simulink model "AcasXuClosedLoop"  (R2019b)
settings: Solver=VariableStepAuto  StartTime=0.0  StopTime=15.0  RelTol=1e-3
libraries: neural x312, simulink x2
(part 1 of 17)
settings Model: Creator=manzand  LastModifiedBy=manzand

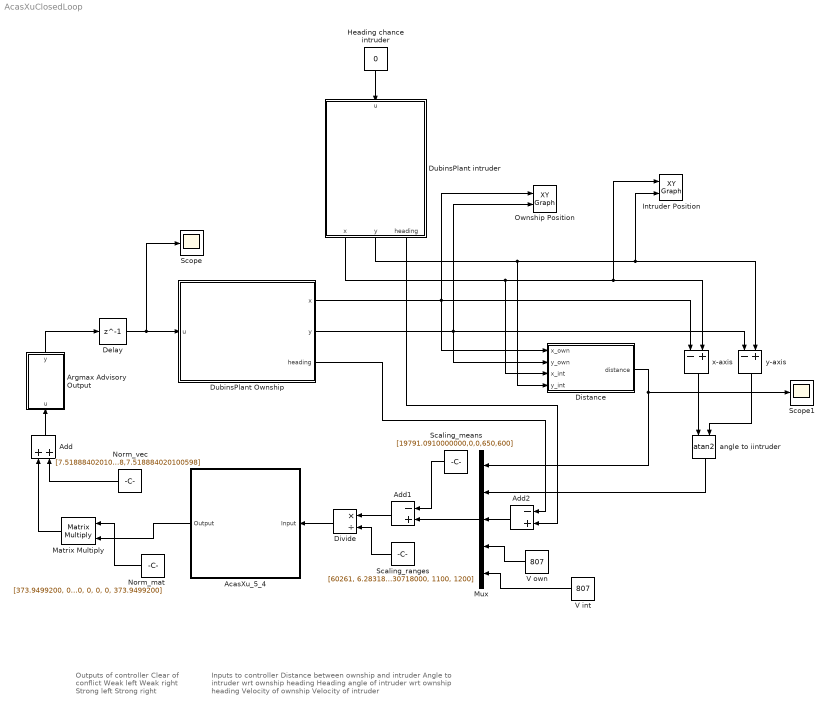
== system AcasXuClosedLoop ==
  note: Outputs of controller
      | Clear of conflict
      | Weak left
      | Weak right
      | Strong left
      | Strong right
  note: Inputs to controller
      | Distance between ownship and intruder
      | Angle to intruder wrt ownship heading
      | Heading angle of intruder wrt ownship heading
      | Velocity of ownship
      | Velocity of intruder
  AcasXu_5_4 : Subsystem  Priority=17
      mask help: Feed-Forward Neural Network
      mask Display: e = 0.06;c1 = [120 150 230]/255;c2 = ([120 150 230]+0)/383;c3 = ([120 150 230]+128)/383;patch([0 1 1 0],[0 0 1 1],c1);patch([0 1 1 1-e 1-e 0+e],[0 0 1 1-e 0+e 0+e],c2);patch([0 0 1 1-e 0+e 0+e],[0 1 1 1-e 1-e 0+e],c3);plot([0 1 1 0 0],[0 0 1 1 0]);fprintf('NNET');port_label('input',1,' Input');port_label('output',1,'Output ');
  Add : Sum  Priority=20
  Add1 : Sum  Priority=14  Inputs=-+
  Add2 : Sum  Priority=9  Inputs=-+
  Argmax Advisory Output : MATLAB Function  Priority=21  TreatAsAtomicUnit=on
  Delay : Delay  Priority=1  DelayLength=1  InitialCondition=0
  Distance : MATLAB Function  Priority=5  TreatAsAtomicUnit=on
  Divide : Product  Priority=16  Inputs=*/
  DubinsPlant Ownship : Stateflow chart  Priority=2  BlockKeywords=__PRM__SERIALIZED__DATA__:Stateflow Chart,Stateflow Diagram  TreatAsAtomicUnit=on
  DubinsPlant intruder : Stateflow chart  Priority=4  BlockKeywords=__PRM__SERIALIZED__DATA__:Stateflow Chart,Stateflow Diagram  TreatAsAtomicUnit=on
  "Heading chance intruder " : Constant  Priority=3  Value=0
  Intruder Position : simulink/Sinks/XY Graph  xmin=800  xmax=1200  ymin=8000  ymax=10000  st=-1
  Matrix Multiply : Product  Priority=19  Multiplication=Matrix(*)
  Mux : Mux  Priority=12  Inputs=5
  Norm_mat : Constant  Priority=18  Value=|  VectorParams1D=off
      | [373.9499200, 0, 0, 0, 0; 0, 373.9499200, 0, 0, 0;
      | 0, 0, 373.9499200, 0, 0;
      | 0, 0, 0, 373.9499200, 0;
      | 0, 0, 0, 0, 373.9499200]
  "Norm_vec " : Constant  Value=[7.518884020100598, 7.518884020100598,7.518884020100598,7.518884020100598,7.518884020100598]
  Ownship Position : simulink/Sinks/XY Graph  xmin=800  xmax=1200  ymin=8000  ymax=10000  st=-1
  Scaling_means : Constant  Priority=13  Value=[19791.0910000000,0,0,650,600]
  Scaling_ranges : Constant  Priority=15  Value=[60261, 6.28318530718000, 6.28318530718000, 1100, 1200]  VectorParams1D=off
  Scope : Scope
  Scope1 : Scope
  V int : Constant  Priority=11  Value=807
  V own : Constant  Priority=10  Value=807
  angle to iintruder : Trigonometry  Priority=8  Operator=atan2  OutputSignalType=real
  x-axis : Sum  Priority=6  Inputs=-+
  y-axis : Sum  Priority=7  Inputs=-+
  wires:
  "Heading chance intruder "/1 -> DubinsPlant intruder/1(u)
  V own/1 -> Mux/4
  V int/1 -> Mux/5
  "Norm_vec "/1 -> Add/2
  AcasXu_5_4/1(Output) -> Matrix Multiply/2
  Matrix Multiply/1 -> Add/1
  Norm_mat/1 -> Matrix Multiply/1
  Add/1 -> Argmax Advisory Output/1(u)
  Argmax Advisory Output/1(y) -> Delay/1
  Scaling_means/1 -> Add1/1
  Mux/1 -> Add1/2
  Add1/1 -> Divide/1
  Divide/1 -> AcasXu_5_4/1(Input)
  Scaling_ranges/1 -> Divide/2
  DubinsPlant Ownship/3(heading) -> Add2/1
  DubinsPlant intruder/3(heading) -> Add2/2
  Add2/1 -> Mux/3
  DubinsPlant Ownship/1(x) -> Ownship Position/1, x-axis/1, Distance/1(x_own)
  DubinsPlant Ownship/2(y) -> Ownship Position/2, y-axis/1, Distance/2(y_own)
  DubinsPlant intruder/1(x) -> Intruder Position/1, x-axis/2, Distance/3(x_int)
  DubinsPlant intruder/2(y) -> Intruder Position/2, y-axis/2, Distance/4(y_int)
  Distance/1(distance) -> Scope1/1, Mux/1
  angle to iintruder/1 -> Mux/2
  y-axis/1 -> angle to iintruder/2
  x-axis/1 -> angle to iintruder/1
  Delay/1 -> Scope/1, DubinsPlant Ownship/1(u)

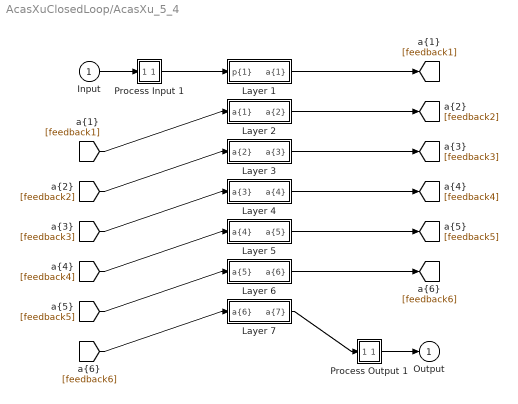
== system AcasXuClosedLoop/AcasXu_5_4 ==
  Input : Inport  PortDimensions=5
      mask Display: e = 0.06;c1 = [120 230 180]/255;c2 = ([120 230 180]+0)/(256+128);c3 = ([120 230 180]+128)/(256+128);patch([0 1 1 0],[0 0 1 1],c1);patch([0 1 1 1-e 1-e 0+e],[0 0 1 1-e 0+e 0+e],c2);patch([0 0 1 1-e 0+e 0+e],[0 1 1 1-e 1-e 0+e],c3);plot([0 1 1 0 0],[0 0 1 1 0]);
  Layer 1 : Subsystem
      mask Display: e = 0.06;c1 = [120 150 230]/255;c2 = ([120 150 230]+0)/383;c3 = ([120 150 230]+128)/383;patch([0 1 1 0],[0 0 1 1],c1);patch([0 1 1 1-e 1-e 0+e],[0 0 1 1-e 0+e 0+e],c2);patch([0 0 1 1-e 0+e 0+e],[0 1 1 1-e 1-e 0+e],c3);plot([0 1 1 0 0],[0 0 1 1 0]);
  Layer 2 : Subsystem
      mask Display: e = 0.06;c1 = [120 150 230]/255;c2 = ([120 150 230]+0)/383;c3 = ([120 150 230]+128)/383;patch([0 1 1 0],[0 0 1 1],c1);patch([0 1 1 1-e 1-e 0+e],[0 0 1 1-e 0+e 0+e],c2);patch([0 0 1 1-e 0+e 0+e],[0 1 1 1-e 1-e 0+e],c3);plot([0 1 1 0 0],[0 0 1 1 0]);
  Layer 3 : Subsystem
      mask Display: e = 0.06;c1 = [120 150 230]/255;c2 = ([120 150 230]+0)/383;c3 = ([120 150 230]+128)/383;patch([0 1 1 0],[0 0 1 1],c1);patch([0 1 1 1-e 1-e 0+e],[0 0 1 1-e 0+e 0+e],c2);patch([0 0 1 1-e 0+e 0+e],[0 1 1 1-e 1-e 0+e],c3);plot([0 1 1 0 0],[0 0 1 1 0]);
  Layer 4 : Subsystem
      mask Display: e = 0.06;c1 = [120 150 230]/255;c2 = ([120 150 230]+0)/383;c3 = ([120 150 230]+128)/383;patch([0 1 1 0],[0 0 1 1],c1);patch([0 1 1 1-e 1-e 0+e],[0 0 1 1-e 0+e 0+e],c2);patch([0 0 1 1-e 0+e 0+e],[0 1 1 1-e 1-e 0+e],c3);plot([0 1 1 0 0],[0 0 1 1 0]);
  Layer 5 : Subsystem
      mask Display: e = 0.06;c1 = [120 150 230]/255;c2 = ([120 150 230]+0)/383;c3 = ([120 150 230]+128)/383;patch([0 1 1 0],[0 0 1 1],c1);patch([0 1 1 1-e 1-e 0+e],[0 0 1 1-e 0+e 0+e],c2);patch([0 0 1 1-e 0+e 0+e],[0 1 1 1-e 1-e 0+e],c3);plot([0 1 1 0 0],[0 0 1 1 0]);
  Layer 6 : Subsystem
      mask Display: e = 0.06;c1 = [120 150 230]/255;c2 = ([120 150 230]+0)/383;c3 = ([120 150 230]+128)/383;patch([0 1 1 0],[0 0 1 1],c1);patch([0 1 1 1-e 1-e 0+e],[0 0 1 1-e 0+e 0+e],c2);patch([0 0 1 1-e 0+e 0+e],[0 1 1 1-e 1-e 0+e],c3);plot([0 1 1 0 0],[0 0 1 1 0]);
  Layer 7 : Subsystem
      mask Display: e = 0.06;c1 = [120 150 230]/255;c2 = ([120 150 230]+0)/383;c3 = ([120 150 230]+128)/383;patch([0 1 1 0],[0 0 1 1],c1);patch([0 1 1 1-e 1-e 0+e],[0 0 1 1-e 0+e 0+e],c2);patch([0 0 1 1-e 0+e 0+e],[0 1 1 1-e 1-e 0+e],c3);plot([0 1 1 0 0],[0 0 1 1 0]);
  Process Input 1 : Subsystem
      mask Display: e = 0.06;c1 = [120 150 230]/255;c2 = ([120 150 230]+0)/383;c3 = ([120 150 230]+128)/383;patch([0 1 1 0],[0 0 1 1],c1);patch([0 1 1 1-e 1-e 0+e],[0 0 1 1-e 0+e 0+e],c2);patch([0 0 1 1-e 0+e 0+e],[0 1 1 1-e 1-e 0+e],c3);plot([0 1 1 0 0],[0 0 1 1 0]);
  Process Output 1 : Subsystem
      mask Display: e = 0.06;c1 = [120 150 230]/255;c2 = ([120 150 230]+0)/383;c3 = ([120 150 230]+128)/383;patch([0 1 1 0],[0 0 1 1],c1);patch([0 1 1 1-e 1-e 0+e],[0 0 1 1-e 0+e 0+e],c2);patch([0 0 1 1-e 0+e 0+e],[0 1 1 1-e 1-e 0+e],c3);plot([0 1 1 0 0],[0 0 1 1 0]);
  Output : Outport  InitialOutput=[0;0;0;0;0]
      mask Display: e = 0.06;c1 = [120 230 180]/255;c2 = ([120 230 180]+0)/(256+128);c3 = ([120 230 180]+128)/(256+128);patch([0 1 1 0],[0 0 1 1],c1);patch([0 1 1 1-e 1-e 0+e],[0 0 1 1-e 0+e 0+e],c2);patch([0 0 1 1-e 0+e 0+e],[0 1 1 1-e 1-e 0+e],c3);plot([0 1 1 0 0],[0 0 1 1 0]);
  wires:
  Input/1 -> Process Input 1/1(x)
  Process Output 1/1(y) -> Output/1
  Process Input 1/1(p) -> Layer 1/1("p{1}")
  Layer 1/1("a{1}") -> [feedback1]
  [feedback1] -> Layer 2/1("a{1} ")
  Layer 2/1("a{2}") -> [feedback2]
  [feedback2] -> Layer 3/1("a{2} ")
  Layer 3/1("a{3}") -> [feedback3]
  [feedback3] -> Layer 4/1("a{3} ")
  Layer 4/1("a{4}") -> [feedback4]
  [feedback4] -> Layer 5/1("a{4} ")
  Layer 5/1("a{5}") -> [feedback5]
  [feedback5] -> Layer 6/1("a{5} ")
  Layer 6/1("a{6}") -> [feedback6]
  [feedback6] -> Layer 7/1("a{6} ")
  Layer 7/1("a{7}") -> Process Output 1/1(a)

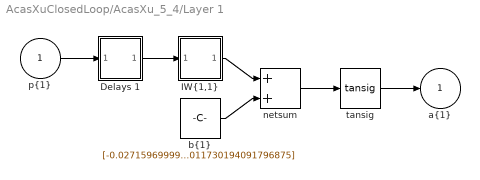
== system AcasXuClosedLoop/AcasXu_5_4/Layer 1 ==
  "p{1}" : Inport  PortDimensions=5
      mask Display: e = 0.06;c1 = [120 230 180]/255;c2 = ([120 230 180]+0)/(256+128);c3 = ([120 230 180]+128)/(256+128);patch([0 1 1 0],[0 0 1 1],c1);patch([0 1 1 1-e 1-e 0+e],[0 0 1 1-e 0+e 0+e],c2);patch([0 0 1 1-e 0+e 0+e],[0 1 1 1-e 1-e 0+e],c3);plot([0 1 1 0 0],[0 0 1 1 0]);
  Delays 1 : Subsystem
      mask Display: e = 0.06;c1 = [120 150 230]/255;c2 = ([120 150 230]+0)/383;c3 = ([120 150 230]+128)/383;patch([0 1 1 0],[0 0 1 1],c1);patch([0 1 1 1-e 1-e 0+e],[0 0 1 1-e 0+e 0+e],c2);patch([0 0 1 1-e 0+e 0+e],[0 1 1 1-e 1-e 0+e],c3);plot([0 1 1 0 0],[0 0 1 1 0]);disp('0');
  "IW{1,1}" : Subsystem
      mask Display: e = 0.06;c1 = [120 150 230]/255;c2 = ([120 150 230]+0)/383;c3 = ([120 150 230]+128)/383;patch([0 1 1 0],[0 0 1 1],c1);patch([0 1 1 1-e 1-e 0+e],[0 0 1 1-e 0+e 0+e],c2);patch([0 0 1 1-e 0+e 0+e],[0 1 1 1-e 1-e 0+e],c3);plot([0 1 1 0 0],[0 0 1 1 0]);disp('W');
  "b{1}" : Constant  Value=[-0.0271596999999999984265475205802431446500122547149658203125;-0.46073100000000000164845914696343243122100830078125;-0.44965500000000002689404254851979203522205352783203125;0.260207999999999994855670593096874654293060302734375;-0.00276675000000000011202150318467829492874443531036376953125;0.4017589999999999772484216009615920484066009521484375;-0.1695399999999999962607688530624727718532085418701171875;0.05863140000000000018332002582610584795475006103515625;0.383875000000000021760371282653068192303180694580078125;-0.57595200000000001949729266925714910030364990234375;0.12246400000000000340971695322878076694905757904052734375;-0.301667999999999991711518987358431331813335418701171875;-0.49515100000000000779465381128829903900623321533203125;0.0887586999999999959332086518770665861666202545166015625;0.294314000000000020040857862113625742495059967041015625;-0.26196099999999999941024952931911684572696685791015625;-0.355347000000000023955948336151777766644954681396484375;-0.02843299999999999994049204588009160943329334259033203125;-0.309130999999999989125143429191666655242443084716796875;-0.4068220000000000169393388205207884311676025390625;-0.2495509999999999950492934885915019549429416656494140625;-0.0188888000000000007283507130750876967795193195343017578125;0.0037677100000000000694366786291311655077151954174041748046875;-0.372257999999999977802644934854470193386077880859375;-0.457145999999999996799004975400748662650585174560546875;0.283702999999999982971843337509199045598506927490234375;-0.473530999999999979710452180370339192450046539306640625;0.1901130000000000042081893525391933508217334747314453125;-0.593428999999999984282794684986583888530731201171875;-0.26313500000000000778044295657309703528881072998046875;-0.041796800000000002006661503628492937423288822174072265625;-0.335610000000000019415580254644737578928470611572265625;-0.287716000000000027281288339509046636521816253662109375;0.042627800000000000413269418686468270607292652130126953125;-0.045651100000000000012079226507921703159809112548828125;-0.33134900000000000463984406451345421373844146728515625;-0.168113000000000012423839734765351749956607818603515625;-0.07636020000000000307327496784637332893908023834228515625;0.004191480000000000032123192994504279340617358684539794921875;0.1780650000000000010569323194431490264832973480224609375;-0.327330999999999983085530175230815075337886810302734375;-0.0216147999999999999853894649959329399280250072479248046875;-0.4477889999999999925961446933797560632228851318359375;0.0291006000000000007721379091663038707338273525238037109375;0.156737999999999988443022402861970476806163787841796875;0.037446899999999998243094267991182277910411357879638671875;0.11496800000000000074873440780720557086169719696044921875;-0.07569610000000000227249330464474041946232318878173828125;0.141199999999999992184029906638897955417633056640625;-0.04411299999999999943423034665102022700011730194091796875]
      mask Display: e = 0.06;c1 = [120 150 230]/255;c2 = ([120 150 230]+0)/383;c3 = ([120 150 230]+128)/383;patch([0 1 1 0],[0 0 1 1],c1);patch([0 1 1 1-e 1-e 0+e],[0 0 1 1-e 0+e 0+e],c2);patch([0 0 1 1-e 0+e 0+e],[0 1 1 1-e 1-e 0+e],c3);plot([0 1 1 0 0],[0 0 1 1 0]);disp('b');
  netsum : Sum  Inputs=2  SaturateOnIntegerOverflow=on  InputSameDT=on  OutDataTypeStr=Inherit: Same as first input
      mask Display: e = 0.06;c1 = [120 150 230]/255;c2 = ([120 150 230]+0)/383;c3 = ([120 150 230]+128)/383;patch([0 1 1 0],[0 0 1 1],c1);patch([0 1 1 1-e 1-e 0+e],[0 0 1 1-e 0+e 0+e],c2);patch([0 0 1 1-e 0+e 0+e],[0 1 1 1-e 1-e 0+e],c3);plot([0 1 1 0 0],[0 0 1 1 0]);disp('+');
  tansig : neural/Transfer Functions/tansig
      settings: SourceProductName=Deep Learning Toolbox
  "a{1}" : Outport  InitialOutput=[0;0;0;0;0;0;0;0;0;0;0;0;0;0;0;0;0;0;0;0;0;0;0;0;0;0;0;0;0;0;0;0;0;0;0;0;0;0;0;0;0;0;0;0;0;0;0;0;0;0]
      mask Display: e = 0.06;c1 = [120 230 180]/255;c2 = ([120 230 180]+0)/(256+128);c3 = ([120 230 180]+128)/(256+128);patch([0 1 1 0],[0 0 1 1],c1);patch([0 1 1 1-e 1-e 0+e],[0 0 1 1-e 0+e 0+e],c2);patch([0 0 1 1-e 0+e 0+e],[0 1 1 1-e 1-e 0+e],c3);plot([0 1 1 0 0],[0 0 1 1 0]);
  wires:
  "p{1}"/1 -> Delays 1/1("p{1}")
  Delays 1/1("pd{1,1}") -> "IW{1,1}"/1("pd{1,1}")
  "IW{1,1}"/1("iz{1,1}") -> netsum/1
  "b{1}"/1 -> netsum/2
  netsum/1 -> tansig/1
  tansig/1 -> "a{1}"/1

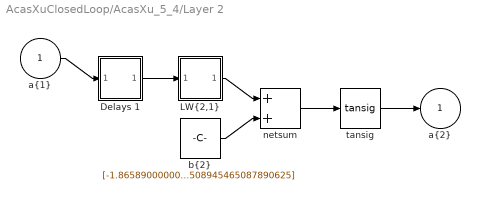
== system AcasXuClosedLoop/AcasXu_5_4/Layer 2 ==
  "a{1} " : Inport  PortDimensions=50
      mask Display: e = 0.06;c1 = [120 230 180]/255;c2 = ([120 230 180]+0)/(256+128);c3 = ([120 230 180]+128)/(256+128);patch([0 1 1 0],[0 0 1 1],c1);patch([0 1 1 1-e 1-e 0+e],[0 0 1 1-e 0+e 0+e],c2);patch([0 0 1 1-e 0+e 0+e],[0 1 1 1-e 1-e 0+e],c3);plot([0 1 1 0 0],[0 0 1 1 0]);
  Delays 1 : Subsystem
      mask Display: e = 0.06;c1 = [120 150 230]/255;c2 = ([120 150 230]+0)/383;c3 = ([120 150 230]+128)/383;patch([0 1 1 0],[0 0 1 1],c1);patch([0 1 1 1-e 1-e 0+e],[0 0 1 1-e 0+e 0+e],c2);patch([0 0 1 1-e 0+e 0+e],[0 1 1 1-e 1-e 0+e],c3);plot([0 1 1 0 0],[0 0 1 1 0]);disp('0');
  "LW{2,1}" : Subsystem
      mask Display: e = 0.06;c1 = [120 150 230]/255;c2 = ([120 150 230]+0)/383;c3 = ([120 150 230]+128)/383;patch([0 1 1 0],[0 0 1 1],c1);patch([0 1 1 1-e 1-e 0+e],[0 0 1 1-e 0+e 0+e],c2);patch([0 0 1 1-e 0+e 0+e],[0 1 1 1-e 1-e 0+e],c3);plot([0 1 1 0 0],[0 0 1 1 0]);disp('W');
  "b{2}" : Constant  Value=[-1.8658900000000000485300688524148426949977874755859375;-1.063120000000000064943606048473156988620758056640625;-0.425429000000000001602273869139025919139385223388671875;-0.97161600000000003518607627484016120433807373046875;-0.2178299999999999958522067800004151649773120880126953125;-0.78610700000000000020605739337042905390262603759765625;0.01303039999999999927482452477534025092609226703643798828125;-0.5963030000000000274695821644854731857776641845703125;-0.06148649999999999948840923025272786617279052734375;1.2156800000000000938626953939092345535755157470703125;-1.0417300000000000448352466264623217284679412841796875;-0.0189298000000000000986322135076989070512354373931884765625;0.996596999999999955122120809392072260379791259765625;0.478447000000000011166179092469974420964717864990234375;-0.50230600000000003024780426130746491253376007080078125;1.379129999999999967030817060731351375579833984375;-0.00918792000000000046167070166802659514360129833221435546875;0.6292940000000000200230942937196232378482818603515625;-0.294291000000000024794388764348695985972881317138671875;-0.76959999999999995079491554861306212842464447021484375;-0.309201000000000003620215238697710447013378143310546875;-0.314163000000000025568880346327205188572406768798828125;0.6841180000000000038795633372501470148563385009765625;-0.434860999999999997545074847948853857815265655517578125;-0.0129557999999999999551913987261286820285022258758544921875;0.64022900000000004805400521945557557046413421630859375;-1.0621300000000000185451654033386148512363433837890625;0.67218699999999997896082959414343349635601043701171875;-0.95618099999999994764721122919581830501556396484375;0.7149499999999999744204615126363933086395263671875;0.33513599999999998946265122867771424353122711181640625;-0.158001000000000002554401135057560168206691741943359375;0.55337899999999995426236409912235103547573089599609375;-0.71827600000000002555822220529080368578433990478515625;-1.685820000000000096207486421917565166950225830078125;-1.41626999999999991786125974613241851329803466796875;-0.05192270000000000218509654814624809660017490386962890625;-0.01547459999999999981368237200740622938610613346099853515625;-0.10283499999999999585664767209891579113900661468505859375;-0.01436939999999999918733895043487791554071009159088134765625;-0.314643999999999979255704829483875073492527008056640625;-0.05589399999999999923971927273669280111789703369140625;-0.34012100000000000665778543407213874161243438720703125;-0.231157000000000001360689338980591855943202972412109375;-0.66548499999999999321431687349104322493076324462890625;-0.31501699999999999146638174352119676768779754638671875;-0.0191915000000000002255973186038318090140819549560546875;-0.5179139999999999854907173357787542045116424560546875;-0.9061099999999999710098563809879124164581298828125;-0.007343360000000000165076841085465275682508945465087890625]
      mask Display: e = 0.06;c1 = [120 150 230]/255;c2 = ([120 150 230]+0)/383;c3 = ([120 150 230]+128)/383;patch([0 1 1 0],[0 0 1 1],c1);patch([0 1 1 1-e 1-e 0+e],[0 0 1 1-e 0+e 0+e],c2);patch([0 0 1 1-e 0+e 0+e],[0 1 1 1-e 1-e 0+e],c3);plot([0 1 1 0 0],[0 0 1 1 0]);disp('b');
  netsum : Sum  Inputs=2  SaturateOnIntegerOverflow=on  InputSameDT=on  OutDataTypeStr=Inherit: Same as first input
      mask Display: e = 0.06;c1 = [120 150 230]/255;c2 = ([120 150 230]+0)/383;c3 = ([120 150 230]+128)/383;patch([0 1 1 0],[0 0 1 1],c1);patch([0 1 1 1-e 1-e 0+e],[0 0 1 1-e 0+e 0+e],c2);patch([0 0 1 1-e 0+e 0+e],[0 1 1 1-e 1-e 0+e],c3);plot([0 1 1 0 0],[0 0 1 1 0]);disp('+');
  tansig : neural/Transfer Functions/tansig
      settings: SourceProductName=Deep Learning Toolbox
  "a{2}" : Outport  InitialOutput=[0;0;0;0;0;0;0;0;0;0;0;0;0;0;0;0;0;0;0;0;0;0;0;0;0;0;0;0;0;0;0;0;0;0;0;0;0;0;0;0;0;0;0;0;0;0;0;0;0;0]
      mask Display: e = 0.06;c1 = [120 230 180]/255;c2 = ([120 230 180]+0)/(256+128);c3 = ([120 230 180]+128)/(256+128);patch([0 1 1 0],[0 0 1 1],c1);patch([0 1 1 1-e 1-e 0+e],[0 0 1 1-e 0+e 0+e],c2);patch([0 0 1 1-e 0+e 0+e],[0 1 1 1-e 1-e 0+e],c3);plot([0 1 1 0 0],[0 0 1 1 0]);
  wires:
  "a{1} "/1 -> Delays 1/1("p{2}")
  Delays 1/1("pd{2,1}") -> "LW{2,1}"/1("ad{2,1}")
  "LW{2,1}"/1("lz{2,1}") -> netsum/1
  "b{2}"/1 -> netsum/2
  netsum/1 -> tansig/1
  tansig/1 -> "a{2}"/1

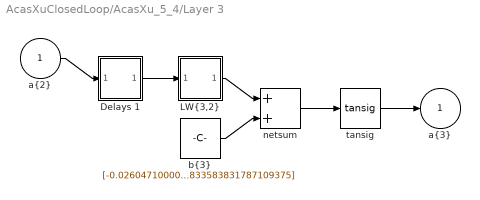
== system AcasXuClosedLoop/AcasXu_5_4/Layer 3 ==
  "a{2} " : Inport  PortDimensions=50
      mask Display: e = 0.06;c1 = [120 230 180]/255;c2 = ([120 230 180]+0)/(256+128);c3 = ([120 230 180]+128)/(256+128);patch([0 1 1 0],[0 0 1 1],c1);patch([0 1 1 1-e 1-e 0+e],[0 0 1 1-e 0+e 0+e],c2);patch([0 0 1 1-e 0+e 0+e],[0 1 1 1-e 1-e 0+e],c3);plot([0 1 1 0 0],[0 0 1 1 0]);
  Delays 1 : Subsystem
      mask Display: e = 0.06;c1 = [120 150 230]/255;c2 = ([120 150 230]+0)/383;c3 = ([120 150 230]+128)/383;patch([0 1 1 0],[0 0 1 1],c1);patch([0 1 1 1-e 1-e 0+e],[0 0 1 1-e 0+e 0+e],c2);patch([0 0 1 1-e 0+e 0+e],[0 1 1 1-e 1-e 0+e],c3);plot([0 1 1 0 0],[0 0 1 1 0]);disp('0');
  "LW{3,2}" : Subsystem
      mask Display: e = 0.06;c1 = [120 150 230]/255;c2 = ([120 150 230]+0)/383;c3 = ([120 150 230]+128)/383;patch([0 1 1 0],[0 0 1 1],c1);patch([0 1 1 1-e 1-e 0+e],[0 0 1 1-e 0+e 0+e],c2);patch([0 0 1 1-e 0+e 0+e],[0 1 1 1-e 1-e 0+e],c3);plot([0 1 1 0 0],[0 0 1 1 0]);disp('W');
  "b{3}" : Constant  Value=[-0.0260471000000000001139977001685110735706984996795654296875;-0.95781199999999999672439798814593814313411712646484375;0.06712279999999999635651448670614627189934253692626953125;0.052227400000000000213074002886060043238103389739990234375;-0.80914099999999999912603243501507677137851715087890625;0.051077799999999999591704380463852430693805217742919921875;-0.44884800000000002473399263180908747017383575439453125;-0.28515699999999999381117277152952738106250762939453125;0.78063300000000002132338750016060657799243927001953125;0.092305899999999996285993120181956328451633453369140625;0.416785000000000016573409311604336835443973541259765625;-0.025808299999999999296829145123410853557288646697998046875;-0.32824500000000000898836560736526735126972198486328125;0.574192000000000035697667044587433338165283203125;-0.304387000000000018662404954739031381905078887939453125;0.298094999999999998863131622783839702606201171875;-0.1890969999999999873185885235216119326651096343994140625;-1.2466699999999999448618837050162255764007568359375;-1.39599999999999990762944435118697583675384521484375;-3.188289999999999846380660528666339814662933349609375;-0.27131600000000000161293201017542742192745208740234375;-0.2078069999999999917239534852342330850660800933837890625;-0.8511450000000000404298816647497005760669708251953125;-0.5834799999999999986499688020558096468448638916015625;-2.492529999999999912319026407203637063503265380859375;-0.06499770000000000547135670103671145625412464141845703125;0.6484330000000000371329633708228357136249542236328125;-0.07179760000000000308428838025065488182008266448974609375;-0.50401700000000004830980060432921163737773895263671875;-0.82203800000000004644107320928014814853668212890625;-0.03150820000000000009610090501155355013906955718994140625;1.32204999999999994741983755375258624553680419921875;-0.020012200000000000821298584696705802343785762786865234375;1.1339200000000000390087961932295002043247222900390625;-0.2227639999999999897983826713243615813553333282470703125;-0.391488000000000002653877118063974194228649139404296875;0.7049549999999999982946974341757595539093017578125;-0.399880999999999986460608170091290958225727081298828125;1.90359999999999995878852132591418921947479248046875;-0.07875959999999999905373471165148657746613025665283203125;0.059131200000000001815170236341145937331020832061767578125;-0.986048999999999953303131405846215784549713134765625;-0.51995299999999999851496568226139061152935028076171875;0.54076500000000005119460411151521839201450347900390625;-1.46724999999999994315658113919198513031005859375;-0.27974799999999999666755456928513012826442718505859375;-0.391129999999999977688958097132854163646697998046875;-0.01308740000000000076874062671095089172013103961944580078125;-0.378466000000000024616753080408670939505100250244140625;-0.7134519999999999750883716842508874833583831787109375]
      mask Display: e = 0.06;c1 = [120 150 230]/255;c2 = ([120 150 230]+0)/383;c3 = ([120 150 230]+128)/383;patch([0 1 1 0],[0 0 1 1],c1);patch([0 1 1 1-e 1-e 0+e],[0 0 1 1-e 0+e 0+e],c2);patch([0 0 1 1-e 0+e 0+e],[0 1 1 1-e 1-e 0+e],c3);plot([0 1 1 0 0],[0 0 1 1 0]);disp('b');
  netsum : Sum  Inputs=2  SaturateOnIntegerOverflow=on  InputSameDT=on  OutDataTypeStr=Inherit: Same as first input
      mask Display: e = 0.06;c1 = [120 150 230]/255;c2 = ([120 150 230]+0)/383;c3 = ([120 150 230]+128)/383;patch([0 1 1 0],[0 0 1 1],c1);patch([0 1 1 1-e 1-e 0+e],[0 0 1 1-e 0+e 0+e],c2);patch([0 0 1 1-e 0+e 0+e],[0 1 1 1-e 1-e 0+e],c3);plot([0 1 1 0 0],[0 0 1 1 0]);disp('+');
  tansig : neural/Transfer Functions/tansig
      settings: SourceProductName=Deep Learning Toolbox
  "a{3}" : Outport  InitialOutput=[0;0;0;0;0;0;0;0;0;0;0;0;0;0;0;0;0;0;0;0;0;0;0;0;0;0;0;0;0;0;0;0;0;0;0;0;0;0;0;0;0;0;0;0;0;0;0;0;0;0]
      mask Display: e = 0.06;c1 = [120 230 180]/255;c2 = ([120 230 180]+0)/(256+128);c3 = ([120 230 180]+128)/(256+128);patch([0 1 1 0],[0 0 1 1],c1);patch([0 1 1 1-e 1-e 0+e],[0 0 1 1-e 0+e 0+e],c2);patch([0 0 1 1-e 0+e 0+e],[0 1 1 1-e 1-e 0+e],c3);plot([0 1 1 0 0],[0 0 1 1 0]);
  wires:
  "a{2} "/1 -> Delays 1/1("p{3}")
  Delays 1/1("pd{3,2}") -> "LW{3,2}"/1("ad{3,2}")
  "LW{3,2}"/1("lz{3,2}") -> netsum/1
  "b{3}"/1 -> netsum/2
  netsum/1 -> tansig/1
  tansig/1 -> "a{3}"/1

== system AcasXuClosedLoop/AcasXu_5_4/Layer 4 ==
  "a{3} " : Inport  PortDimensions=50
      mask Display: e = 0.06;c1 = [120 230 180]/255;c2 = ([120 230 180]+0)/(256+128);c3 = ([120 230 180]+128)/(256+128);patch([0 1 1 0],[0 0 1 1],c1);patch([0 1 1 1-e 1-e 0+e],[0 0 1 1-e 0+e 0+e],c2);patch([0 0 1 1-e 0+e 0+e],[0 1 1 1-e 1-e 0+e],c3);plot([0 1 1 0 0],[0 0 1 1 0]);
  Delays 1 : Subsystem
      mask Display: e = 0.06;c1 = [120 150 230]/255;c2 = ([120 150 230]+0)/383;c3 = ([120 150 230]+128)/383;patch([0 1 1 0],[0 0 1 1],c1);patch([0 1 1 1-e 1-e 0+e],[0 0 1 1-e 0+e 0+e],c2);patch([0 0 1 1-e 0+e 0+e],[0 1 1 1-e 1-e 0+e],c3);plot([0 1 1 0 0],[0 0 1 1 0]);disp('0');
  "LW{4,3}" : Subsystem
      mask Display: e = 0.06;c1 = [120 150 230]/255;c2 = ([120 150 230]+0)/383;c3 = ([120 150 230]+128)/383;patch([0 1 1 0],[0 0 1 1],c1);patch([0 1 1 1-e 1-e 0+e],[0 0 1 1-e 0+e 0+e],c2);patch([0 0 1 1-e 0+e 0+e],[0 1 1 1-e 1-e 0+e],c3);plot([0 1 1 0 0],[0 0 1 1 0]);disp('W');
  "b{4}" : Constant  Value=[0.92520400000000002638245177877251990139484405517578125;0.485126000000000001666222715357434935867786407470703125;-0.807425999999999977063680489663966000080108642578125;-2.15824000000000015830892152735032141208648681640625;0.278378000000000014324541552923619747161865234375;-0.010241699999999999415312146311407559551298618316650390625;1.5972699999999999675992512493394315242767333984375;1.1845000000000001083577672034152783453464508056640625;0.292349000000000025512036927466397173702716827392578125;0.254375000000000017763568394002504646778106689453125;-0.92610000000000003428368700042483396828174591064453125;-1.109760000000000079722894952283240854740142822265625;-1.3649999999999999911182158029987476766109466552734375;1.547940000000000093649532573181204497814178466796875;-1.1489700000000000468247662865906022489070892333984375;-2.696709999999999940456518743303604423999786376953125;0.269450000000000022826185386293218471109867095947265625;-0.50999600000000000488142859467188827693462371826171875;-0.0417912000000000005695000027117202989757061004638671875;-3.870779999999999887450030655600130558013916015625;-0.05673229999999999939586103891997481696307659149169921875;0.290472999999999981213250066502951085567474365234375;0.69952800000000003866063025270705111324787139892578125;-0.1625040000000000095514707254551467485725879669189453125;-1.7176400000000000556354962100158445537090301513671875;-1.379610000000000002984279490192420780658721923828125;-0.06355270000000000363282737225745222531259059906005859375;-1.2160200000000001008260142043582163751125335693359375;0.050255199999999999871391764827421866357326507568359375;-0.36520900000000000584776671530562452971935272216796875;-1.926369999999999915729631538852117955684661865234375;-1.115699999999999914024328973027877509593963623046875;-0.249817000000000011272760502833989448845386505126953125;-3.32918000000000002813749233609996736049652099609375;-0.77362100000000000310507175527163781225681304931640625;0.06598089999999999510915671407929039560258388519287109375;-1.4626900000000000456878979093744419515132904052734375;0.3062110000000000109565689854207448661327362060546875;0.0796802000000000065771388335633673705160617828369140625;-3.39552999999999993718802215880714356899261474609375;-0.6837940000000000129176669361186213791370391845703125;-2.03028999999999992809307514107786118984222412109375;-2.202780000000000182325265996041707694530487060546875;0.97622200000000003417000016270321793854236602783203125;0.42702899999999999192112909440766088664531707763671875;-0.373614999999999974900077859274460934102535247802734375;-0.038825100000000001276845296160900034010410308837890625;3.00532999999999983486986820935271680355072021484375;-0.51424999999999998490096686509787105023860931396484375;-2.690119999999999844675357962842099368572235107421875]
      mask Display: e = 0.06;c1 = [120 150 230]/255;c2 = ([120 150 230]+0)/383;c3 = ([120 150 230]+128)/383;patch([0 1 1 0],[0 0 1 1],c1);patch([0 1 1 1-e 1-e 0+e],[0 0 1 1-e 0+e 0+e],c2);patch([0 0 1 1-e 0+e 0+e],[0 1 1 1-e 1-e 0+e],c3);plot([0 1 1 0 0],[0 0 1 1 0]);disp('b');
  netsum : Sum  Inputs=2  SaturateOnIntegerOverflow=on  InputSameDT=on  OutDataTypeStr=Inherit: Same as first input
      mask Display: e = 0.06;c1 = [120 150 230]/255;c2 = ([120 150 230]+0)/383;c3 = ([120 150 230]+128)/383;patch([0 1 1 0],[0 0 1 1],c1);patch([0 1 1 1-e 1-e 0+e],[0 0 1 1-e 0+e 0+e],c2);patch([0 0 1 1-e 0+e 0+e],[0 1 1 1-e 1-e 0+e],c3);plot([0 1 1 0 0],[0 0 1 1 0]);disp('+');
  tansig : neural/Transfer Functions/tansig
      settings: SourceProductName=Deep Learning Toolbox
  "a{4}" : Outport  InitialOutput=[0;0;0;0;0;0;0;0;0;0;0;0;0;0;0;0;0;0;0;0;0;0;0;0;0;0;0;0;0;0;0;0;0;0;0;0;0;0;0;0;0;0;0;0;0;0;0;0;0;0]
      mask Display: e = 0.06;c1 = [120 230 180]/255;c2 = ([120 230 180]+0)/(256+128);c3 = ([120 230 180]+128)/(256+128);patch([0 1 1 0],[0 0 1 1],c1);patch([0 1 1 1-e 1-e 0+e],[0 0 1 1-e 0+e 0+e],c2);patch([0 0 1 1-e 0+e 0+e],[0 1 1 1-e 1-e 0+e],c3);plot([0 1 1 0 0],[0 0 1 1 0]);
  wires:
  "a{3} "/1 -> Delays 1/1("p{4}")
  Delays 1/1("pd{4,3}") -> "LW{4,3}"/1("ad{4,3}")
  "LW{4,3}"/1("lz{4,3}") -> netsum/1
  "b{4}"/1 -> netsum/2
  netsum/1 -> tansig/1
  tansig/1 -> "a{4}"/1

== system AcasXuClosedLoop/AcasXu_5_4/Layer 5 ==
  "a{4} " : Inport  PortDimensions=50
      mask Display: e = 0.06;c1 = [120 230 180]/255;c2 = ([120 230 180]+0)/(256+128);c3 = ([120 230 180]+128)/(256+128);patch([0 1 1 0],[0 0 1 1],c1);patch([0 1 1 1-e 1-e 0+e],[0 0 1 1-e 0+e 0+e],c2);patch([0 0 1 1-e 0+e 0+e],[0 1 1 1-e 1-e 0+e],c3);plot([0 1 1 0 0],[0 0 1 1 0]);
  Delays 1 : Subsystem
      mask Display: e = 0.06;c1 = [120 150 230]/255;c2 = ([120 150 230]+0)/383;c3 = ([120 150 230]+128)/383;patch([0 1 1 0],[0 0 1 1],c1);patch([0 1 1 1-e 1-e 0+e],[0 0 1 1-e 0+e 0+e],c2);patch([0 0 1 1-e 0+e 0+e],[0 1 1 1-e 1-e 0+e],c3);plot([0 1 1 0 0],[0 0 1 1 0]);disp('0');
  "LW{5,4}" : Subsystem
      mask Display: e = 0.06;c1 = [120 150 230]/255;c2 = ([120 150 230]+0)/383;c3 = ([120 150 230]+128)/383;patch([0 1 1 0],[0 0 1 1],c1);patch([0 1 1 1-e 1-e 0+e],[0 0 1 1-e 0+e 0+e],c2);patch([0 0 1 1-e 0+e 0+e],[0 1 1 1-e 1-e 0+e],c3);plot([0 1 1 0 0],[0 0 1 1 0]);disp('W');
  "b{5}" : Constant  Value=[0.972806999999999977291054165107198059558868408203125;-2.491659999999999985931253831950016319751739501953125;0.20180100000000000814992517916834913194179534912109375;-1.0420899999999999607780409860424697399139404296875;1.0066900000000000847677483761799521744251251220703125;-0.9243900000000000449773551736143417656421661376953125;-0.0250631000000000013494538819713852717541158199310302734375;0.463849000000000011301182212264393456280231475830078125;0.7509580000000000143955958264996297657489776611328125;0.2153090000000000003854694341498543508350849151611328125;-1.771030000000000104165565062430687248706817626953125;1.0371099999999999763389268991886638104915618896484375;-2.087079999999999824211727172951214015483856201171875;1.783300000000000107291953099775128066539764404296875;-0.01392419999999999942474904202072139014489948749542236328125;0.303771999999999986474819024806492961943149566650390625;-0.60735799999999995346655623507103882730007171630859375;1.6324099999999999166533370953402481973171234130859375;0.757519999999999971151964928139932453632354736328125;-0.29550799999999999290167806975659914314746856689453125;-0.7769340000000000134861011247267015278339385986328125;1.3666400000000000769517782828188501298427581787109375;0.9245309999999999917008608463220298290252685546875;-3.20005000000000006110667527536861598491668701171875;0.463500999999999996337152197156683541834354400634765625;-0.89910699999999998954791635696892626583576202392578125;1.2499100000000000765254526413627900183200836181640625;0.255919000000000007588596417917869985103607177734375;0.75380599999999997606892065959982573986053466796875;1.267889999999999961488583721802569925785064697265625;0.33895799999999998153299429759499616920948028564453125;0.67463799999999995993249513048795051872730255126953125;-1.425710000000000032827074392116628587245941162109375;-1.5239000000000000323296944770845584571361541748046875;0.2496549999999999880362366866393131203949451446533203125;-1.9637100000000000665778543407213874161243438720703125;0.1005189999999999972413178284114110283553600311279296875;1.5726800000000000778754838393069803714752197265625;0.10919900000000000439559499909591977484524250030517578125;0.18748799999999998799893319301190786063671112060546875;-1.1184600000000000097344354799133725464344024658203125;-0.56281499999999995420552068026154302060604095458984375;-2.27423000000000019582557797548361122608184814453125;-1.9608200000000000073896444519050419330596923828125;-0.397635000000000016218137943724286742508411407470703125;0.45664599999999999635491576555068604648113250732421875;0.1645230000000000025739410602909629233181476593017578125;0.9636160000000000280806489172391593456268310546875;-0.2931690000000000129176669361186213791370391845703125;-2.208979999999999943582906780648045241832733154296875]
      mask Display: e = 0.06;c1 = [120 150 230]/255;c2 = ([120 150 230]+0)/383;c3 = ([120 150 230]+128)/383;patch([0 1 1 0],[0 0 1 1],c1);patch([0 1 1 1-e 1-e 0+e],[0 0 1 1-e 0+e 0+e],c2);patch([0 0 1 1-e 0+e 0+e],[0 1 1 1-e 1-e 0+e],c3);plot([0 1 1 0 0],[0 0 1 1 0]);disp('b');
  netsum : Sum  Inputs=2  SaturateOnIntegerOverflow=on  InputSameDT=on  OutDataTypeStr=Inherit: Same as first input
      mask Display: e = 0.06;c1 = [120 150 230]/255;c2 = ([120 150 230]+0)/383;c3 = ([120 150 230]+128)/383;patch([0 1 1 0],[0 0 1 1],c1);patch([0 1 1 1-e 1-e 0+e],[0 0 1 1-e 0+e 0+e],c2);patch([0 0 1 1-e 0+e 0+e],[0 1 1 1-e 1-e 0+e],c3);plot([0 1 1 0 0],[0 0 1 1 0]);disp('+');
  tansig : neural/Transfer Functions/tansig
      settings: SourceProductName=Deep Learning Toolbox
  "a{5}" : Outport  InitialOutput=[0;0;0;0;0;0;0;0;0;0;0;0;0;0;0;0;0;0;0;0;0;0;0;0;0;0;0;0;0;0;0;0;0;0;0;0;0;0;0;0;0;0;0;0;0;0;0;0;0;0]
      mask Display: e = 0.06;c1 = [120 230 180]/255;c2 = ([120 230 180]+0)/(256+128);c3 = ([120 230 180]+128)/(256+128);patch([0 1 1 0],[0 0 1 1],c1);patch([0 1 1 1-e 1-e 0+e],[0 0 1 1-e 0+e 0+e],c2);patch([0 0 1 1-e 0+e 0+e],[0 1 1 1-e 1-e 0+e],c3);plot([0 1 1 0 0],[0 0 1 1 0]);
  wires:
  "a{4} "/1 -> Delays 1/1("p{5}")
  Delays 1/1("pd{5,4}") -> "LW{5,4}"/1("ad{5,4}")
  "LW{5,4}"/1("lz{5,4}") -> netsum/1
  "b{5}"/1 -> netsum/2
  netsum/1 -> tansig/1
  tansig/1 -> "a{5}"/1

== system AcasXuClosedLoop/AcasXu_5_4/Layer 6 ==
  "a{5} " : Inport  PortDimensions=50
      mask Display: e = 0.06;c1 = [120 230 180]/255;c2 = ([120 230 180]+0)/(256+128);c3 = ([120 230 180]+128)/(256+128);patch([0 1 1 0],[0 0 1 1],c1);patch([0 1 1 1-e 1-e 0+e],[0 0 1 1-e 0+e 0+e],c2);patch([0 0 1 1-e 0+e 0+e],[0 1 1 1-e 1-e 0+e],c3);plot([0 1 1 0 0],[0 0 1 1 0]);
  Delays 1 : Subsystem
      mask Display: e = 0.06;c1 = [120 150 230]/255;c2 = ([120 150 230]+0)/383;c3 = ([120 150 230]+128)/383;patch([0 1 1 0],[0 0 1 1],c1);patch([0 1 1 1-e 1-e 0+e],[0 0 1 1-e 0+e 0+e],c2);patch([0 0 1 1-e 0+e 0+e],[0 1 1 1-e 1-e 0+e],c3);plot([0 1 1 0 0],[0 0 1 1 0]);disp('0');
  "LW{6,5}" : Subsystem
      mask Display: e = 0.06;c1 = [120 150 230]/255;c2 = ([120 150 230]+0)/383;c3 = ([120 150 230]+128)/383;patch([0 1 1 0],[0 0 1 1],c1);patch([0 1 1 1-e 1-e 0+e],[0 0 1 1-e 0+e 0+e],c2);patch([0 0 1 1-e 0+e 0+e],[0 1 1 1-e 1-e 0+e],c3);plot([0 1 1 0 0],[0 0 1 1 0]);disp('W');
  "b{6}" : Constant  Value=[-0.03584400000000000086064488868942135013639926910400390625;0.3950919999999999987494447850622236728668212890625;0.81037199999999998123456634857575409114360809326171875;-0.6100820000000000131734623209922574460506439208984375;0.3043810000000000126618715512449853122234344482421875;0.297632999999999980911269403804908506572246551513671875;-0.317309000000000007712941396675887517631053924560546875;0.5944359999999999644160197931341826915740966796875;-0.474615000000000009094947017729282379150390625;-0.042387399999999998689848013100345269776880741119384765625;-0.1414539999999999964064301138932933099567890167236328125;-0.57975699999999996681054881264572031795978546142578125;0.423561999999999994059862729045562446117401123046875;2.110040000000000137703182190307416021823883056640625;0.072345300000000001272582039746339432895183563232421875;0.005821699999999999965150099257016336196102201938629150390625;-2.23111000000000014864554032101295888423919677734375;-0.146581999999999990080823408789001405239105224609375;0.11111400000000000443112213588392478413879871368408203125;0.97744500000000000827782287160516716539859771728515625;0.1338229999999999975113240680002490989863872528076171875;-0.07875649999999999317790155828333809040486812591552734375;-0.043342600000000001958522233280746149830520153045654296875;0.01344509999999999975972553301062362152151763439178466796875;-0.1041789999999999938307126967629301361739635467529296875;0.0262880999999999982741361037597016547806560993194580078125;0.63892800000000005145039949638885445892810821533203125;0.325452999999999992297716744360513985157012939453125;-0.79462600000000005451283868751488626003265380859375;2.42914999999999992041921359486877918243408203125;-1.1207599999999999784705551064689643681049346923828125;-1.3263700000000000489563944938709028065204620361328125;-0.96074999999999999289457264239899814128875732421875;1.569630000000000080717654782347381114959716796875;0.0757612000000000007648992550457478500902652740478515625;0.36353699999999999903366187936626374721527099609375;-1.0098599999999999798916405779891647398471832275390625;-0.673143000000000046867398850736208260059356689453125;0.035201599999999999557331875621457584202289581298828125;-0.4322369999999999823359075890039093792438507080078125;0.5649159999999999737241296315914951264858245849609375;0.1010250000000000036859404417555197142064571380615234375;-1.8055099999999999482724888366647064685821533203125;-0.250587999999999977429609998580417595803737640380859375;0.89383599999999996388311274131410755217075347900390625;-0.3178170000000000161577418111846782267093658447265625;0.123091000000000005965006266706041060388088226318359375;0.251315000000000010604850331219495274126529693603515625;-0.327707000000000026052049406644073314964771270751953125;-1.7915799999999999503330627703689970076084136962890625]
      mask Display: e = 0.06;c1 = [120 150 230]/255;c2 = ([120 150 230]+0)/383;c3 = ([120 150 230]+128)/383;patch([0 1 1 0],[0 0 1 1],c1);patch([0 1 1 1-e 1-e 0+e],[0 0 1 1-e 0+e 0+e],c2);patch([0 0 1 1-e 0+e 0+e],[0 1 1 1-e 1-e 0+e],c3);plot([0 1 1 0 0],[0 0 1 1 0]);disp('b');
  netsum : Sum  Inputs=2  SaturateOnIntegerOverflow=on  InputSameDT=on  OutDataTypeStr=Inherit: Same as first input
      mask Display: e = 0.06;c1 = [120 150 230]/255;c2 = ([120 150 230]+0)/383;c3 = ([120 150 230]+128)/383;patch([0 1 1 0],[0 0 1 1],c1);patch([0 1 1 1-e 1-e 0+e],[0 0 1 1-e 0+e 0+e],c2);patch([0 0 1 1-e 0+e 0+e],[0 1 1 1-e 1-e 0+e],c3);plot([0 1 1 0 0],[0 0 1 1 0]);disp('+');
  tansig : neural/Transfer Functions/tansig
      settings: SourceProductName=Deep Learning Toolbox
  "a{6}" : Outport  InitialOutput=[0;0;0;0;0;0;0;0;0;0;0;0;0;0;0;0;0;0;0;0;0;0;0;0;0;0;0;0;0;0;0;0;0;0;0;0;0;0;0;0;0;0;0;0;0;0;0;0;0;0]
      mask Display: e = 0.06;c1 = [120 230 180]/255;c2 = ([120 230 180]+0)/(256+128);c3 = ([120 230 180]+128)/(256+128);patch([0 1 1 0],[0 0 1 1],c1);patch([0 1 1 1-e 1-e 0+e],[0 0 1 1-e 0+e 0+e],c2);patch([0 0 1 1-e 0+e 0+e],[0 1 1 1-e 1-e 0+e],c3);plot([0 1 1 0 0],[0 0 1 1 0]);
  wires:
  "a{5} "/1 -> Delays 1/1("p{6}")
  Delays 1/1("pd{6,5}") -> "LW{6,5}"/1("ad{6,5}")
  "LW{6,5}"/1("lz{6,5}") -> netsum/1
  "b{6}"/1 -> netsum/2
  netsum/1 -> tansig/1
  tansig/1 -> "a{6}"/1

== system AcasXuClosedLoop/AcasXu_5_4/Layer 7 ==
  "a{6} " : Inport  PortDimensions=50
      mask Display: e = 0.06;c1 = [120 230 180]/255;c2 = ([120 230 180]+0)/(256+128);c3 = ([120 230 180]+128)/(256+128);patch([0 1 1 0],[0 0 1 1],c1);patch([0 1 1 1-e 1-e 0+e],[0 0 1 1-e 0+e 0+e],c2);patch([0 0 1 1-e 0+e 0+e],[0 1 1 1-e 1-e 0+e],c3);plot([0 1 1 0 0],[0 0 1 1 0]);
  Delays 1 : Subsystem
      mask Display: e = 0.06;c1 = [120 150 230]/255;c2 = ([120 150 230]+0)/383;c3 = ([120 150 230]+128)/383;patch([0 1 1 0],[0 0 1 1],c1);patch([0 1 1 1-e 1-e 0+e],[0 0 1 1-e 0+e 0+e],c2);patch([0 0 1 1-e 0+e 0+e],[0 1 1 1-e 1-e 0+e],c3);plot([0 1 1 0 0],[0 0 1 1 0]);disp('0');
  "LW{7,6}" : Subsystem
      mask Display: e = 0.06;c1 = [120 150 230]/255;c2 = ([120 150 230]+0)/383;c3 = ([120 150 230]+128)/383;patch([0 1 1 0],[0 0 1 1],c1);patch([0 1 1 1-e 1-e 0+e],[0 0 1 1-e 0+e 0+e],c2);patch([0 0 1 1-e 0+e 0+e],[0 1 1 1-e 1-e 0+e],c3);plot([0 1 1 0 0],[0 0 1 1 0]);disp('W');
  "b{7}" : Constant  Value=[-0.0207069000000000003058886477447231300175189971923828125;0.01821319999999999883488754903737572021782398223876953125;-0.0187906000000000010519141113718433189205825328826904296875;0.0188730000000000008864020628607249818742275238037109375;-0.01817169999999999896456159831359400413930416107177734375]
      mask Display: e = 0.06;c1 = [120 150 230]/255;c2 = ([120 150 230]+0)/383;c3 = ([120 150 230]+128)/383;patch([0 1 1 0],[0 0 1 1],c1);patch([0 1 1 1-e 1-e 0+e],[0 0 1 1-e 0+e 0+e],c2);patch([0 0 1 1-e 0+e 0+e],[0 1 1 1-e 1-e 0+e],c3);plot([0 1 1 0 0],[0 0 1 1 0]);disp('b');
  netsum : Sum  Inputs=2  SaturateOnIntegerOverflow=on  InputSameDT=on  OutDataTypeStr=Inherit: Same as first input
      mask Display: e = 0.06;c1 = [120 150 230]/255;c2 = ([120 150 230]+0)/383;c3 = ([120 150 230]+128)/383;patch([0 1 1 0],[0 0 1 1],c1);patch([0 1 1 1-e 1-e 0+e],[0 0 1 1-e 0+e 0+e],c2);patch([0 0 1 1-e 0+e 0+e],[0 1 1 1-e 1-e 0+e],c3);plot([0 1 1 0 0],[0 0 1 1 0]);disp('+');
  purelin : neural/Transfer Functions/purelin
      settings: SourceProductName=Deep Learning Toolbox
  "a{7}" : Outport  InitialOutput=[0;0;0;0;0]
      mask Display: e = 0.06;c1 = [120 230 180]/255;c2 = ([120 230 180]+0)/(256+128);c3 = ([120 230 180]+128)/(256+128);patch([0 1 1 0],[0 0 1 1],c1);patch([0 1 1 1-e 1-e 0+e],[0 0 1 1-e 0+e 0+e],c2);patch([0 0 1 1-e 0+e 0+e],[0 1 1 1-e 1-e 0+e],c3);plot([0 1 1 0 0],[0 0 1 1 0]);
  wires:
  "a{6} "/1 -> Delays 1/1("p{7}")
  Delays 1/1("pd{7,6}") -> "LW{7,6}"/1("ad{7,6}")
  "LW{7,6}"/1("lz{7,6}") -> netsum/1
  "b{7}"/1 -> netsum/2
  netsum/1 -> purelin/1
  purelin/1 -> "a{7}"/1

== system AcasXuClosedLoop/AcasXu_5_4/Process Input 1 ==
  x : Inport  PortDimensions=5
      mask Display: e = 0.06;c1 = [120 230 180]/255;c2 = ([120 230 180]+0)/(256+128);c3 = ([120 230 180]+128)/(256+128);patch([0 1 1 0],[0 0 1 1],c1);patch([0 1 1 1-e 1-e 0+e],[0 0 1 1-e 0+e 0+e],c2);patch([0 0 1 1-e 0+e 0+e],[0 1 1 1-e 1-e 0+e],c3);plot([0 1 1 0 0],[0 0 1 1 0]);
  p : Outport  PortDimensions=5
      mask Display: e = 0.06;c1 = [120 230 180]/255;c2 = ([120 230 180]+0)/(256+128);c3 = ([120 230 180]+128)/(256+128);patch([0 1 1 0],[0 0 1 1],c1);patch([0 1 1 1-e 1-e 0+e],[0 0 1 1-e 0+e 0+e],c2);patch([0 0 1 1-e 0+e 0+e],[0 1 1 1-e 1-e 0+e],c3);plot([0 1 1 0 0],[0 0 1 1 0]);
  wires:
  x/1 -> p/1

== system AcasXuClosedLoop/AcasXu_5_4/Process Output 1 ==
  a : Inport  PortDimensions=5
      mask Display: e = 0.06;c1 = [120 230 180]/255;c2 = ([120 230 180]+0)/(256+128);c3 = ([120 230 180]+128)/(256+128);patch([0 1 1 0],[0 0 1 1],c1);patch([0 1 1 1-e 1-e 0+e],[0 0 1 1-e 0+e 0+e],c2);patch([0 0 1 1-e 0+e 0+e],[0 1 1 1-e 1-e 0+e],c3);plot([0 1 1 0 0],[0 0 1 1 0]);
  y : Outport  PortDimensions=5
      mask Display: e = 0.06;c1 = [120 230 180]/255;c2 = ([120 230 180]+0)/(256+128);c3 = ([120 230 180]+128)/(256+128);patch([0 1 1 0],[0 0 1 1],c1);patch([0 1 1 1-e 1-e 0+e],[0 0 1 1-e 0+e 0+e],c2);patch([0 0 1 1-e 0+e 0+e],[0 1 1 1-e 1-e 0+e],c3);plot([0 1 1 0 0],[0 0 1 1 0]);
  wires:
  a/1 -> y/1

== system AcasXuClosedLoop/AcasXu_5_4/Layer 1/Delays 1 ==
  "p{1}" : Inport  PortDimensions=5
      mask Display: e = 0.06;c1 = [120 230 180]/255;c2 = ([120 230 180]+0)/(256+128);c3 = ([120 230 180]+128)/(256+128);patch([0 1 1 0],[0 0 1 1],c1);patch([0 1 1 1-e 1-e 0+e],[0 0 1 1-e 0+e 0+e],c2);patch([0 0 1 1-e 0+e 0+e],[0 1 1 1-e 1-e 0+e],c3);plot([0 1 1 0 0],[0 0 1 1 0]);
  mux : Mux  Inputs=1
      mask Display: e = 0.06;c1 = [120 150 230]/255;c2 = ([120 150 230]+0)/383;c3 = ([120 150 230]+128)/383;patch([0 1 1 0],[0 0 1 1],c1);patch([0 1 1 1-e 1-e 0+e],[0 0 1 1-e 0+e 0+e],c2);patch([0 0 1 1-e 0+e 0+e],[0 1 1 1-e 1-e 0+e],c3);plot([0 1 1 0 0],[0 0 1 1 0]);disp('Mux')
  "pd{1,1}" : Outport
      mask Display: e = 0.06;c1 = [120 230 180]/255;c2 = ([120 230 180]+0)/(256+128);c3 = ([120 230 180]+128)/(256+128);patch([0 1 1 0],[0 0 1 1],c1);patch([0 1 1 1-e 1-e 0+e],[0 0 1 1-e 0+e 0+e],c2);patch([0 0 1 1-e 0+e 0+e],[0 1 1 1-e 1-e 0+e],c3);plot([0 1 1 0 0],[0 0 1 1 0]);
  wires:
  "p{1}"/1 -> mux/1
  mux/1 -> "pd{1,1}"/1
